simulink model "FidelityStepResponse"  (R2021b)
settings: configuration reference "ctrlConfigSet" (kept outside this file)
undefined symbols (not defined in the file): aircraftTmax, ap, DiscIntNeverNeededParam, Earth, env, initialThrottle, midFidelityUAV, sensors, TFinal, trimT, uavParam, WGS84
libraries: simulink x21, mbdriLib x20, aerolibconvert2 x2, aerolibtransform2 x1, uavalgslib x1
(part 2 of 2)

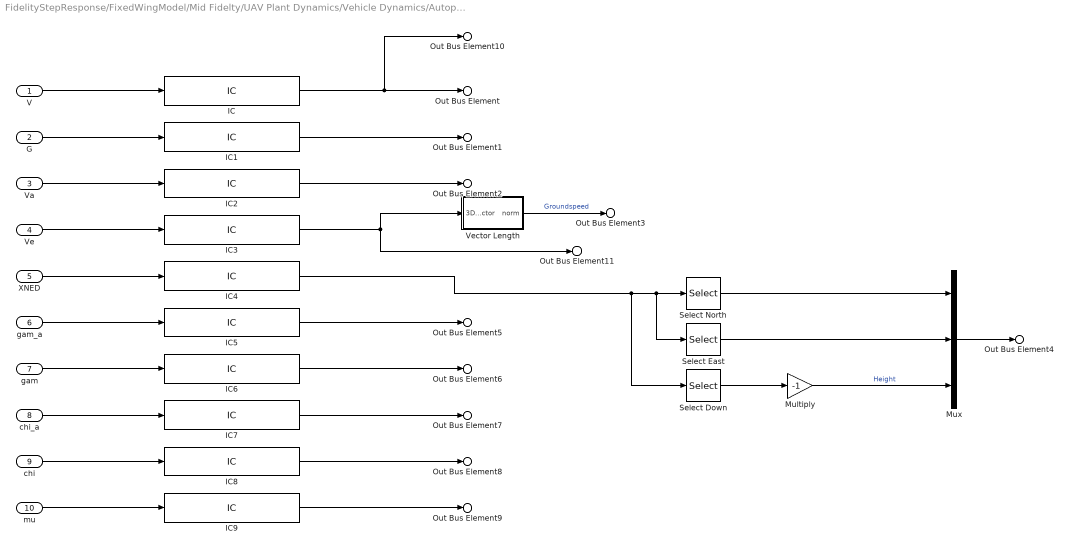
== system FidelityStepResponse/FixedWingModel/Mid Fidelty/UAV Plant Dynamics/Vehicle Dynamics/AutopilotStates ==
  V : Inport
  G : Inport  Port=2
  Va : Inport  Port=3
  Ve : Inport  Port=4
  XNED : Inport  Port=5
  gam_a : Inport  Port=6
  gam : Inport  Port=7
  chi_a : Inport  Port=8
  chi : Inport  Port=9
  mu : Inport  Port=10
  IC : InitialCondition  Value=midFidelityUAV.initialAirspeed
  IC1 : InitialCondition  Value=midFidelityUAV.initialAirspeed
  IC2 : InitialCondition  Value=[midFidelityUAV.initialAirspeed 0 0]
  IC3 : InitialCondition  Value=[midFidelityUAV.initialAirspeed 0 0 ]
  IC4 : InitialCondition  Value=[midFidelityUAV.initialNorth midFidelityUAV.initialEast -midFidelityUAV.initialAltitude]
  IC5 : InitialCondition  Value=midFidelityUAV.initialFlightPathAngle
  IC6 : InitialCondition  Value=midFidelityUAV.initialFlightPathAngle
  IC7 : InitialCondition  Value=midFidelityUAV.initialHeadingAngle
  IC8 : InitialCondition  Value=midFidelityUAV.initialHeadingAngle
  IC9 : InitialCondition  Value=0
  Multiply : Gain  Gain=-1
  Mux : Mux  Inputs=3
  Select Down : Selector  InputPortWidth=3  IndexOptions=Index vector (dialog)  Indices=[3]  OutputSizes=1
  Select East : Selector  InputPortWidth=3  IndexOptions=Index vector (dialog)  Indices=[2]  OutputSizes=1
  Select North : Selector  InputPortWidth=3  IndexOptions=Index vector (dialog)  Indices=[1]  OutputSizes=1
  Vector Length : Subsystem
  Out Bus Element : Outport  PortName=AutopilotStates  Element=V
  Out Bus Element1 : Outport  PortName=AutopilotStates  Element=G
  Out Bus Element2 : Outport  PortName=AutopilotStates  Element=Va
  Out Bus Element3 : Outport  PortName=AutopilotStates  Element=GS
  Out Bus Element4 : Outport  PortName=AutopilotStates  Element=Xe
  Out Bus Element5 : Outport  PortName=AutopilotStates  Element=gamma_a
  Out Bus Element6 : Outport  PortName=AutopilotStates  Element=gamma
  Out Bus Element7 : Outport  PortName=AutopilotStates  Element=chi_a
  Out Bus Element8 : Outport  PortName=AutopilotStates  Element=chi
  Out Bus Element9 : Outport  PortName=AutopilotStates  Element=mu
  Out Bus Element10 : Outport  PortName=AutopilotStates  Element=ias
  Out Bus Element11 : Outport  PortName=AutopilotStates  Element=Ve
  wires:
  IC8/1 -> Out Bus Element8/1
  mu/1 -> IC9/1
  Vector Length/1(norm) -> Out Bus Element3/1  "Groundspeed"
  V/1 -> IC/1
  IC/1 -> Out Bus Element/1, Out Bus Element10/1
  G/1 -> IC1/1
  Va/1 -> IC2/1
  Ve/1 -> IC3/1
  XNED/1 -> IC4/1
  gam_a/1 -> IC5/1
  gam/1 -> IC6/1
  chi_a/1 -> IC7/1
  chi/1 -> IC8/1
  IC1/1 -> Out Bus Element1/1
  IC2/1 -> Out Bus Element2/1
  IC3/1 -> Vector Length/1(3DVector), Out Bus Element11/1
  IC4/1 -> Select Down/1, Select East/1, Select North/1
  IC5/1 -> Out Bus Element5/1
  IC6/1 -> Out Bus Element6/1
  IC7/1 -> Out Bus Element7/1
  Select Down/1 -> Multiply/1
  Select North/1 -> Mux/1
  Select East/1 -> Mux/2
  Multiply/1 -> Mux/3  "Height"
  Mux/1 -> Out Bus Element4/1
  IC9/1 -> Out Bus Element9/1

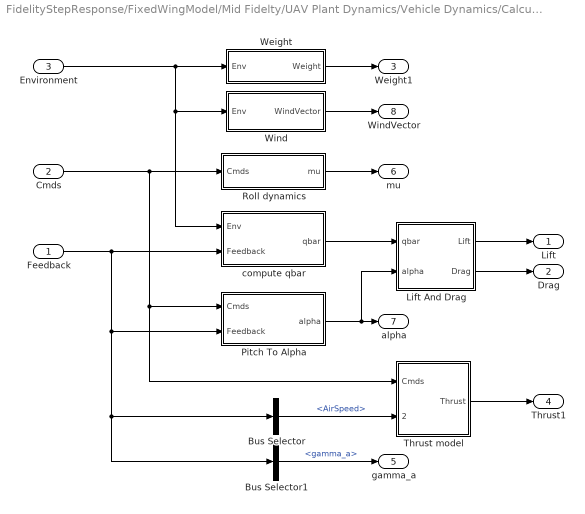
== system FidelityStepResponse/FixedWingModel/Mid Fidelty/UAV Plant Dynamics/Vehicle Dynamics/Calculate Forces ==
  Feedback : Inport
  Cmds : Inport  Port=2
  Environment : Inport  Port=3
  Bus Selector : BusSelector  OutputSignals=AirSpeed
  Bus Selector1 : BusSelector  OutputSignals=gamma_a
  Lift And Drag : Subsystem
  Pitch To Alpha : Subsystem
  Roll dynamics : Subsystem
  Thrust model : Subsystem  Variant=on  VariantControlMode=label  VariantControl=Choice  LabelModeActiveChoice=ThrustAd==1
  Weight : Subsystem
  Wind : Subsystem
  compute qbar : Subsystem
  Lift : Outport
  Drag : Outport  Port=2
  Weight1 : Outport  Port=3
  Thrust1 : Outport  Port=4
  gamma_a : Outport  Port=5
  mu : Outport  Port=6
  alpha : Outport  Port=7
  WindVector : Outport  Port=8
  wires:
  Thrust model/1(Thrust) -> Thrust1/1
  Lift And Drag/1(Lift) -> Lift/1
  Lift And Drag/2(Drag) -> Drag/1
  Wind/1(WindVector) -> WindVector/1
  Bus Selector/1 -> Thrust model/2(Airspeed)  "<AirSpeed>"
  compute qbar/1(qbar) -> Lift And Drag/1(qbar)
  Weight/1(Weight) -> Weight1/1
  Roll dynamics/1(mu) -> mu/1
  Bus Selector1/1 -> gamma_a/1  "<gamma_a>"
  Environment/1 -> compute qbar/1(Env), Wind/1(Env), Weight/1(Env)
  Cmds/1 -> Thrust model/1(Cmds), Pitch To Alpha/1(Cmds), Roll dynamics/1(Cmds)
  Feedback/1 -> Bus Selector/1, Bus Selector1/1, Pitch To Alpha/2(Feedback), compute qbar/2(Feedback)
  Pitch To Alpha/1(alpha) -> alpha/1, Lift And Drag/2(alpha)

== system FidelityStepResponse/FixedWingModel/Mid Fidelty/UAV Plant Dynamics/Vehicle Dynamics/Feedback ==
  In Bus Element : Inport  PortName=AutopilotStates  Element=G
  In Bus Element1 : Inport  PortName=AutopilotStates  Element=V
  In Bus Element2 : Inport  PortName=AutopilotStates  Element=gamma_a
  Out Bus Element : Outport  PortName=Feedback  Element=GroundSpeed
  Out Bus Element1 : Outport  PortName=Feedback  Element=AirSpeed
  Out Bus Element2 : Outport  PortName=Feedback  Element=gamma_a
  wires:
  In Bus Element2/1 -> Out Bus Element2/1
  In Bus Element1/1 -> Out Bus Element1/1
  In Bus Element/1 -> Out Bus Element/1

== system FidelityStepResponse/FixedWingModel/Mid Fidelty/UAV Plant Dynamics/asbState to uavState/Rename chi ==
  In1 : Inport
  Out1 : Outport
  wires:
  In1/1 -> Out1/1

== system FidelityStepResponse/FixedWingModel/Mid Fidelty/UAV Plant Dynamics/asbState to uavState/Rename gamma ==
  In1 : Inport
  Out1 : Outport
  wires:
  In1/1 -> Out1/1

== system FidelityStepResponse/FixedWingModel/Mid Fidelty/UAV Plant Dynamics/asbState to uavState/Rename mu ==
  In1 : Inport
  Out1 : Outport
  wires:
  In1/1 -> Out1/1

== system FidelityStepResponse/FixedWingModel/Mid Fidelty/UAV Plant Dynamics/asbState to uavState/Vector Length ==
  3DVector : Inport
  Add : Sum  Inputs=+
  Square : Math  Operator=square  SaturateOnIntegerOverflow=on
  Square Root : Sqrt  SaturateOnIntegerOverflow=on
  norm : Outport
  wires:
  Square Root/1 -> norm/1
  Add/1 -> Square Root/1
  Square/1 -> Add/1
  3DVector/1 -> Square/1

== system FidelityStepResponse/FixedWingModel/High Fidelty/Autopilot/Inner Loop Autopilot/Latch Trim Conditions/Latch Control Surfaces Trim from any mode ==
  ctrlSurfaces : Inport
  Trigger : TriggerPort  TriggerType=falling  VariantControl=Variant
  Trim : Outport  VectorParamsAs1DForOutWhenUnconnected=off
  wires:
  ctrlSurfaces/1 -> Trim/1

== system FidelityStepResponse/FixedWingModel/High Fidelty/Autopilot/Inner Loop Autopilot/Pitch Controller/Compute Feed Forward ==
  dEFFGain : Inport
  SensorData : Inport  Port=2
  1D Discrete Filter : mbdriLib/Filtering/1D Discrete Filter  bw=10  TSample=ap.apSampleTime
      settings: AttributesFormatString=Fc = 10
  Add5 : Sum  Inputs=+-  OutDataTypeStr=single
  Bus Selector : BusSelector  OutputSignals=Euler
  Constant2 : Constant  OutDataTypeStr=single
      settings: AttributesFormatString=%<Value>
  Constant4 : Constant  OutDataTypeStr=single
      settings: AttributesFormatString=%<Value>
  Product : Product  Inputs=*/  RndMeth=Zero
  Product1 : Product  RndMeth=Zero
  Selector : Selector  InputPortWidth=3  IndexOptions=Index vector (dialog)  Indices=[1]  OutputSizes=1
  Trigonometric Function : Trigonometry  Operator=cos
  "[-60 60]" : Saturate  UpperLimit=60  LowerLimit=-60
      settings: AttributesFormatString="[%<LowerLimit>  %<UpperLimit>]"
  FF : Outport  VectorParamsAs1DForOutWhenUnconnected=off
  wires:
  Selector/1 -> 1D Discrete Filter/1
  Product/1 -> Add5/1
  Constant4/1 -> Product/1
  1D Discrete Filter/1 -> "[-60 60]"/1
  Trigonometric Function/1 -> Product/2
  Constant2/1 -> Add5/2
  Product1/1 -> FF/1
  Add5/1 -> Product1/2
  "[-60 60]"/1 -> Trigonometric Function/1
  Bus Selector/1 -> Selector/1  "<Euler>"
  dEFFGain/1 -> Product1/1
  SensorData/1 -> Bus Selector/1

== system FidelityStepResponse/FixedWingModel/High Fidelty/Sensor Module/Position Filter/Get Vn Ve/Subsystem5 ==
  u : Inport
  Trigonometric Function : Trigonometry
  Trigonometric Function1 : Trigonometry  Operator=cos
  sin(u) : Outport  VectorParamsAs1DForOutWhenUnconnected=off
  cos(u) : Outport  Port=2  VectorParamsAs1DForOutWhenUnconnected=off
  wires:
  u/1 -> Trigonometric Function/1, Trigonometric Function1/1
  Trigonometric Function/1 -> sin(u)/1
  Trigonometric Function1/1 -> cos(u)/1

== system FidelityStepResponse/FixedWingModel/High Fidelty/Sensor Module/Position Filter/Position&Velocity Filter/CompRateOnly ==
  LoPass : Inport
  Gain : Gain  Gain=omega
      settings: AttributesFormatString=%<Gain>
  Sum1 : Sum  Inputs=|+-
  Unit Delay : UnitDelay  SampleTime=T  HasFrameUpgradeWarning=on
  ZPK 1D Discrete Filter : mbdriLib/Filtering/ZPK 1D Discrete Filter  zval=[]  pval=[0]  kval=1  TSample=0.01
  Rate_hat : Outport  VectorParamsAs1DForOutWhenUnconnected=off
  wires:
  Unit Delay/1 -> Sum1/2
  LoPass/1 -> Sum1/1
  Sum1/1 -> Gain/1
  Gain/1 -> ZPK 1D Discrete Filter/1, Rate_hat/1
  ZPK 1D Discrete Filter/1 -> Unit Delay/1

== system FidelityStepResponse/FixedWingModel/High Fidelty/Sensor Module/Position Filter/Position&Velocity Filter/Deriv  ==
  y : Inport
  Gain2 : Gain  Gain=[ 1/(5*ap.apSampleTime) ]
      settings: AttributesFormatString=%<Gain>
  Integer Delay1 : Delay  DelayLength=5  InitialCondition=0  SampleTime=ap.apSampleTime
  Sum5 : Sum  Inputs=-+|
  ydot : Outport  VectorParamsAs1DForOutWhenUnconnected=off
  wires:
  Gain2/1 -> ydot/1
  y/1 -> Integer Delay1/1, Sum5/2
  Integer Delay1/1 -> Sum5/1
  Sum5/1 -> Gain2/1

== system FidelityStepResponse/FixedWingModel/High Fidelty/Sensor Module/Position Filter/Position&Velocity Filter/VN Ve Filter ==
  Vn : Inport
  Ve : Inport  Port=2
  New GPS : Inport  Port=3
  Enable : EnablePort
  Constant : Constant  Value=ap.apSampleTime
      settings: AttributesFormatString=%<Value>
  RateAid for GPS : mbdriLib/Filtering/RateAid for GPS  SystemSampleTime=-1  VariantActivationTime=update diagram  Latency=0  AutoFrameSizeCalculation=off
  RateAid for GPS1 : mbdriLib/Filtering/RateAid for GPS  SystemSampleTime=-1  VariantActivationTime=update diagram  Latency=0  AutoFrameSizeCalculation=off
  Vn_fil : Outport  OutputWhenDisabled=reset  InitialOutput=0  VectorParamsAs1DForOutWhenUnconnected=off
  Ve_fil : Outport  Port=2  OutputWhenDisabled=reset  InitialOutput=0  VectorParamsAs1DForOutWhenUnconnected=off
  wires:
  Constant/1 -> RateAid for GPS1/3, RateAid for GPS/3
  New GPS/1 -> RateAid for GPS/2, RateAid for GPS1/2
  Vn/1 -> RateAid for GPS/1
  Ve/1 -> RateAid for GPS1/1
  RateAid for GPS/1 -> Vn_fil/1
  RateAid for GPS1/1 -> Ve_fil/1

== system FidelityStepResponse/FixedWingModel/High Fidelty/Sensor Module/Position Filter/Position&Velocity Filter/Z Comp Filter ==
  note: Lizarraga, Mariano I. Autonomous landing system for a UAV . Master's Thesis. Monterey California. Naval Postgraduate School, 2004.
  Az : Inport
  Baro Alt : Inport  Port=2
  Xe_z_ic : Inport  Port=3
  Constant : Constant  Value=env.ISA_g  OutDataTypeStr=single
      settings: AttributesFormatString=%<Value>
  Discrete-Time Integrator : DiscreteIntegrator  gainval=1  SampleTime=-1  ICPrevOutput=DiscIntNeverNeededParam  ICPrevScaledInput=DiscIntNeverNeededParam
  Discrete-Time Integrator1 : DiscreteIntegrator  gainval=1  SampleTime=-1  ICPrevOutput=DiscIntNeverNeededParam  ICPrevScaledInput=DiscIntNeverNeededParam
  Discrete-Time Integrator2 : DiscreteIntegrator  gainval=1  InitialConditionSource=external  SampleTime=-1  ICPrevOutput=DiscIntNeverNeededParam  ICPrevScaledInput=DiscIntNeverNeededParam
  Gain : Gain  Gain=21  OutDataTypeStr=single
      settings: AttributesFormatString=%<Gain>
  Gain1 : Gain  Gain=9  OutDataTypeStr=single
      settings: AttributesFormatString=%<Gain>
  Gain2 : Gain  Gain=15  OutDataTypeStr=single
      settings: AttributesFormatString=%<Gain>
  Sum : Sum  Inputs=|++
  Sum1 : Sum  Inputs=+++
  Sum2 : Sum  Inputs=-+|
  Sum3 : Sum  Inputs=|++
  Xe_Z_hat : Outport  VectorParamsAs1DForOutWhenUnconnected=off
  wires:
  Discrete-Time Integrator2/1 -> Sum2/1, Xe_Z_hat/1
  Gain2/1 -> Sum3/2
  Gain1/1 -> Discrete-Time Integrator/1
  Gain/1 -> Sum1/3
  Sum2/1 -> Gain2/1, Gain/1, Gain1/1
  Sum3/1 -> Discrete-Time Integrator2/1
  Discrete-Time Integrator1/1 -> Sum3/1
  Baro Alt/1 -> Sum2/2
  Xe_z_ic/1 -> Discrete-Time Integrator2/2
  Sum1/1 -> Discrete-Time Integrator1/1
  Sum/1 -> Sum1/1
  Discrete-Time Integrator/1 -> Sum1/2
  Constant/1 -> Sum/2
  Az/1 -> Sum/1

== system FidelityStepResponse/FixedWingModel/Mid Fidelty/UAV Plant Dynamics/Vehicle Dynamics/AutopilotStates/Vector Length ==
  3DVector : Inport
  Add : Sum  Inputs=+
  Square : Math  Operator=square  SaturateOnIntegerOverflow=on
  Square Root : Sqrt  SaturateOnIntegerOverflow=on
  norm : Outport
  wires:
  Square Root/1 -> norm/1
  Add/1 -> Square Root/1
  Square/1 -> Add/1
  3DVector/1 -> Square/1

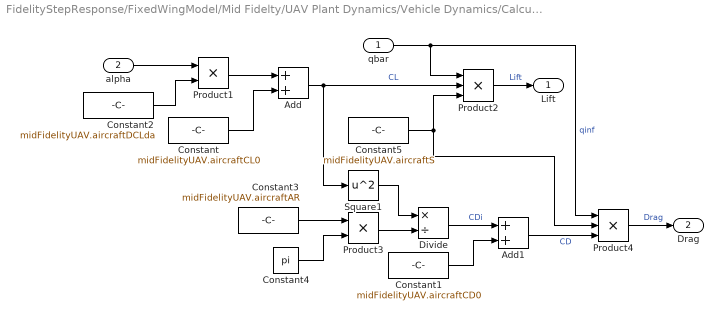
== system FidelityStepResponse/FixedWingModel/Mid Fidelty/UAV Plant Dynamics/Vehicle Dynamics/Calculate Forces/Lift And Drag ==
  qbar : Inport
  alpha : Inport  Port=2
  Add : Sum
  Add1 : Sum
  Constant : Constant  Value=midFidelityUAV.aircraftCL0
  Constant1 : Constant  Value=midFidelityUAV.aircraftCD0
  Constant2 : Constant  Value=midFidelityUAV.aircraftDCLda
  Constant3 : Constant  Value=midFidelityUAV.aircraftAR
  Constant4 : Constant  Value=pi
  Constant5 : Constant  Value=midFidelityUAV.aircraftS
  Divide : Product  Inputs=*/
  Product1 : Product
  Product2 : Product  Inputs=3
  Product3 : Product
  Product4 : Product  Inputs=3
  Square1 : Math  Operator=square  SaturateOnIntegerOverflow=on
  Lift : Outport
  Drag : Outport  Port=2
  wires:
  qbar/1 -> Product4/1, Product2/1  "qinf"
  alpha/1 -> Product1/1
  Constant2/1 -> Product1/2
  Product1/1 -> Add/1
  Constant/1 -> Add/2
  Add/1 -> Product2/2, Square1/1  "CL"
  Constant5/1 -> Product2/3, Product4/2
  Product2/1 -> Lift/1  "Lift"
  Constant3/1 -> Product3/1
  Constant4/1 -> Product3/2
  Product3/1 -> Divide/2
  Square1/1 -> Divide/1
  Divide/1 -> Add1/1  "CDi"
  Constant1/1 -> Add1/2
  Add1/1 -> Product4/3  "CD"
  Product4/1 -> Drag/1  "Drag"

== system FidelityStepResponse/FixedWingModel/Mid Fidelty/UAV Plant Dynamics/Vehicle Dynamics/Calculate Forces/Pitch To Alpha ==
  note: Pitch=alpha+gamma_a
  Cmds : Inport
  Feedback : Inport  Port=2
  Add : Sum  Inputs=+-
  Bus Selector : BusSelector  OutputSignals=Pitch
  Bus Selector1 : BusSelector  OutputSignals=gamma_a
  alpha : Outport
  wires:
  Add/1 -> alpha/1
  Bus Selector1/1 -> Add/2  "<gamma_a>"
  Feedback/1 -> Bus Selector1/1
  Bus Selector/1 -> Add/1  "<Pitch>"
  Cmds/1 -> Bus Selector/1

== system FidelityStepResponse/FixedWingModel/Mid Fidelty/UAV Plant Dynamics/Vehicle Dynamics/Calculate Forces/Roll dynamics ==
  Cmds : Inport
  Bus Selector1 : BusSelector  OutputSignals=Roll
  Saturation2 : Saturate  UpperLimit=midFidelityUAV.maxroll/180*pi  LowerLimit=-midFidelityUAV.maxroll/180*pi
  Transfer Fcn1 : TransferFcn  Numerator=5.448  Denominator=[1 4.6668 5.448]
  mu : Outport
  wires:
  Bus Selector1/1 -> Transfer Fcn1/1  "<Roll>"
  Cmds/1 -> Bus Selector1/1
  Saturation2/1 -> mu/1
  Transfer Fcn1/1 -> Saturation2/1

== system FidelityStepResponse/FixedWingModel/Mid Fidelty/UAV Plant Dynamics/Vehicle Dynamics/Calculate Forces/Thrust model ==
  Cmds : Inport
  Airspeed : Inport  Port=2
  Advanced : Subsystem  VariantControl=ThrustAd==1
  "Simple " : Subsystem  VariantControl=ThrustAd==0
  Thrust : Outport

== system FidelityStepResponse/FixedWingModel/Mid Fidelty/UAV Plant Dynamics/Vehicle Dynamics/Calculate Forces/Weight ==
  Env : Inport
  Bus Selector : BusSelector  OutputSignals=Gravity
  Constant1 : Constant  Value=midFidelityUAV.aircraftM
  Product : Product
  Weight : Outport
  wires:
  Bus Selector/1 -> Product/1  "<Gravity>"
  Constant1/1 -> Product/2
  Product/1 -> Weight/1
  Env/1 -> Bus Selector/1

== system FidelityStepResponse/FixedWingModel/Mid Fidelty/UAV Plant Dynamics/Vehicle Dynamics/Calculate Forces/Wind ==
  Env : Inport
  Bus Creator1 : BusCreator  Inputs=3
  Bus Selector1 : BusSelector  OutputSignals=WindNorth,WindEast,WindDown
  Bus to Vector : BusToVector
  WindVector : Outport
  wires:
  Env/1 -> Bus Selector1/1
  Bus Selector1/3 -> Bus Creator1/3  "<WindDown>"
  Bus Selector1/2 -> Bus Creator1/2  "<WindEast>"
  Bus Selector1/1 -> Bus Creator1/1  "<WindNorth>"
  Bus Creator1/1 -> Bus to Vector/1
  Bus to Vector/1 -> WindVector/1

== system FidelityStepResponse/FixedWingModel/Mid Fidelty/UAV Plant Dynamics/Vehicle Dynamics/Calculate Forces/compute qbar ==
  Env : Inport
  Feedback : Inport  Port=2
  Bus Selector : BusSelector  OutputSignals=Density
  Bus Selector1 : BusSelector  OutputSignals=AirSpeed
  Product7 : Product  Inputs=3
  Square : Math  Operator=square  SaturateOnIntegerOverflow=on
  a : Constant  Value=0.5
  qbar : Outport  OutDataTypeStr=double  PortDimensions=1
  wires:
  Bus Selector1/1 -> Square/1  "<AirSpeed>"
  Feedback/1 -> Bus Selector1/1
  Product7/1 -> qbar/1
  Bus Selector/1 -> Product7/1  "<Density>"
  Env/1 -> Bus Selector/1
  a/1 -> Product7/3
  Square/1 -> Product7/2

== system FidelityStepResponse/FixedWingModel/Mid Fidelty/UAV Plant Dynamics/Vehicle Dynamics/Calculate Forces/Thrust model/Advanced ==
  Airspeed : Inport
  Cmds : Inport  Port=2
  Bus Selector : BusSelector  OutputSignals=Throttle
  Get To : Subsystem
  Mass Conversion : aerolibconvert2/Mass Conversion  IU=lbm  OU=kg
      settings: SourceProductBaseCode=AE
  Mux : Mux  Inputs=2
  Thrust Available (lbs) : Fcn  Expr=u(1) - 0.047*sqrt(u(1))*u(2)
  kg2N : Gain  Gain=9.8065  SaturateOnIntegerOverflow=on  OutDataTypeStr=Inherit: Same as input  ParamDataTypeStr=Inherit: Same as input
      settings: AttributesFormatString=%<Gain>
  Thrust : Outport  Unit=kg*m/s^2  VectorParamsAs1DForOutWhenUnconnected=off
  wires:
  Cmds/1 -> Bus Selector/1
  Bus Selector/1 -> Get To/1(dt)  "<Throttle>"
  Get To/1(To) -> Mux/1
  Mux/1 -> Thrust Available (lbs)/1
  Thrust Available (lbs)/1 -> Mass Conversion/1
  Airspeed/1 -> Mux/2
  kg2N/1 -> Thrust/1
  Mass Conversion/1 -> kg2N/1

== system FidelityStepResponse/FixedWingModel/Mid Fidelty/UAV Plant Dynamics/Vehicle Dynamics/Calculate Forces/Thrust model/Simple  ==
  Cmds : Inport
  Airspeed : Inport  Port=2
  Bus Selector : BusSelector  OutputSignals=throttle_c
  Constant1 : Constant  Value=aircraftTmax
  IC1 : InitialCondition  Value=trimT
  IC7 : InitialCondition  Commented=on  Value=initialThrottle*aircraftTmax
  Product : Product
  Scope : Scope
  Terminator : Terminator
  Thrust : Outport
  wires:
  Airspeed/1 -> Terminator/1
  Bus Selector/1 -> Product/1  "<throttle_c>"
  IC1/1 -> Thrust/1
  Cmds/1 -> Bus Selector/1
  Constant1/1 -> Product/2
  Product/1 -> IC1/1, Scope/1

== system FidelityStepResponse/FixedWingModel/Mid Fidelty/UAV Plant Dynamics/Vehicle Dynamics/Calculate Forces/Thrust model/Advanced/Get To ==
  dt : Inport
  Divide : Product  Inputs=3
  Math Function : Math  Operator=pow  SignedPower=on  SaturateOnIntegerOverflow=on
  Math Function1 : Math  Operator=pow  SignedPower=on  SaturateOnIntegerOverflow=on
  MaxRPM : Gain  Gain=7200  SaturateOnIntegerOverflow=on  OutDataTypeStr=Inherit: Same as input  ParamDataTypeStr=Inherit: Same as input
      settings: AttributesFormatString=%<Gain>
  MaxRPM1 : Gain  Gain=midFidelityUAV.Tfact  SaturateOnIntegerOverflow=on  OutDataTypeStr=Inherit: Same as input  ParamDataTypeStr=Inherit: Same as input
      settings: AttributesFormatString=%<Gain>
  Min RPM : Constant  Value=2000
      settings: AttributesFormatString=%<Value>
  Min Th K : Constant  Value=midFidelityUAV.MinThk
      settings: AttributesFormatString=%<Value>
  Prop Diameter (in) : Constant  Value=17
      settings: AttributesFormatString=%<Value>
  Prop Diameter (in)1 : Constant  Value=2
      settings: AttributesFormatString=%<Value>
  Prop Diameter (in)2 : Constant  Value=4
      settings: AttributesFormatString=%<Value>
  Saturation : Saturate  UpperLimit=1.0  LowerLimit=0
      settings: AttributesFormatString="[%<LowerLimit>  %<UpperLimit>]"
  Sum : Sum  Inputs=|++
  Sum1 : Sum  Inputs=|++
  Th K : Gain  Gain=midFidelityUAV.Thk  SaturateOnIntegerOverflow=on  OutDataTypeStr=Inherit: Same as input  ParamDataTypeStr=Inherit: Same as input
      settings: AttributesFormatString=%<Gain>
  To Constant : Constant  Value=2.83e-12
      settings: AttributesFormatString=%<Value>
  To : Outport  VectorParamsAs1DForOutWhenUnconnected=off
  wires:
  Saturation/1 -> Th K/1
  Prop Diameter (in)1/1 -> Math Function/2
  Prop Diameter (in)2/1 -> Math Function1/2
  Prop Diameter (in)/1 -> Math Function1/1
  Math Function/1 -> Divide/1
  Math Function1/1 -> Divide/2
  To Constant/1 -> Divide/3
  Divide/1 -> MaxRPM1/1
  MaxRPM1/1 -> To/1
  Sum/1 -> Math Function/1
  Min RPM/1 -> Sum/2
  MaxRPM/1 -> Sum/1
  Th K/1 -> Sum1/1
  dt/1 -> Saturation/1
  Sum1/1 -> MaxRPM/1
  Min Th K/1 -> Sum1/2
